simulink model "PAM_Sandbox"  (R2022a)
settings: Solver=VariableStepAuto  StartTime=0.0  StopTime=50  RelTol=1e-3
undefined symbols (not defined in the file or in its folder): m_sandbag, pressure_input, time
libraries: fl_lib x16, nesl_utility x6, SimscapeFluids_lib x1
(part 2 of 2)

== matlab function PAM_Sandbox/MATLAB Function ==
  data: t input; pq output; p input; tq input
function pq = interpolate_pressure(t,p,tq)

pq = interp1(t,p,tq,'linear','extrap');
